simulink model "relay_oscillation"  (R2023a)
settings: Solver=FixedStepAuto  StartTime=0.0  StopTime=15.0  FixedStep=0.01  RelTol=1e-3
settings Model: Creator=Mmoha  LastModifiedBy=Mmoha

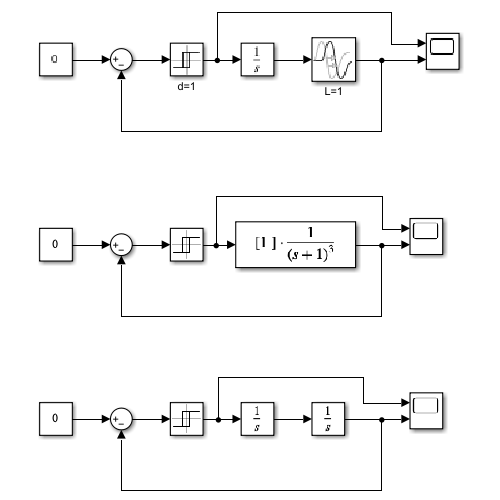
[thumbnail: Simulink's stored preview of the top-level diagram]
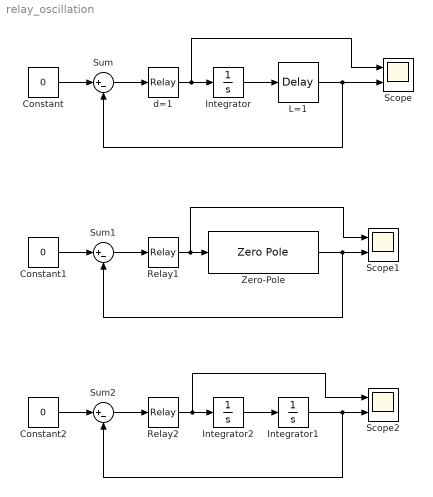
== system relay_oscillation ==
  Constant : Constant  Value=0
  Constant1 : Constant  Value=0
  Constant2 : Constant  Value=0
  Integrator : Integrator
  Integrator1 : Integrator
  Integrator2 : Integrator
  L=1 : TransportDelay
  Relay1 : Relay  OffOutputValue=-1
  Relay2 : Relay  OffOutputValue=-1
  Scope : Scope  NumInputPorts=2
  Scope1 : Scope  NumInputPorts=2
  Scope2 : Scope  NumInputPorts=2
  Sum : Sum  Inputs=|+-
  Sum1 : Sum  Inputs=|+-
  Sum2 : Sum  Inputs=|+-
  Zero-Pole : ZeroPole  Zeros=[]  Poles=[-1 -1 -1]
  d=1 : Relay  OffOutputValue=-1
  wires:
  Integrator/1 -> L=1/1
  L=1/1 -> Sum/2, Scope/2
  d=1/1 -> Scope/1, Integrator/1
  Sum/1 -> d=1/1
  Constant/1 -> Sum/1
  Constant1/1 -> Sum1/1
  Sum1/1 -> Relay1/1
  Relay1/1 -> Scope1/1, Zero-Pole/1
  Zero-Pole/1 -> Scope1/2, Sum1/2
  Integrator2/1 -> Integrator1/1
  Integrator1/1 -> Scope2/2, Sum2/2
  Relay2/1 -> Scope2/1, Integrator2/1
  Sum2/1 -> Relay2/1
  Constant2/1 -> Sum2/1
